simulink model "MotorGenerador_2016"  (Simulink 8.8)
settings: Solver=FixedStepAuto  StartTime=0.0  StopTime=inf  RelTol=1e-3  EnableMultiTasking=on
undefined symbols (not defined in the file or in its folder): sigbuilder_block
libraries: arduinolib x2, simulink x1
settings Model: Creator=Sergio  LastModifiedBy=Sergio  SimulationMode=external  ExtModeTrigDuration=2
settings DataIOCC: LimitDataPoints=off  SaveFormat=Dataset  SignalLoggingSaveFormat=Dataset
settings OptimizationCC: EnhancedBackFolding=on  PassReuseOutputArgsAs=Individual arguments  ZeroExternalMemoryAtStartup=off  ZeroInternalMemoryAtStartup=off  LifeSpan=auto  MaxStackSize=64
settings DebuggingCC: UnderspecifiedInitializationDetection=Simplified  MergeDetectMultiDrivingBlocksExec=error  ParameterTunabilityLossMsg=error  FcnCallInpInsideContextMsg=error  StateNameClashWarn=none  SFUnexpectedBacktrackingDiag=error  SFNoUnconditionalDefaultTransitionDiag=error  SFExecutionAtInitializationDiag=warning  SFMachineParentedDataDiag=error
settings HardwareCC: ProdBitPerInt=16  ProdBitPerPointer=16  ProdBitPerSizeT=16  ProdBitPerPtrDiffT=16  ProdIntDivRoundTo=Zero  ProdEndianess=LittleEndian  ProdWordSize=8  ProdHWDeviceType=Atmel->AVR
settings ModelReferenceCC: PropagateSignalLabelsOutOfModel=on
settings SFSimCC: SimUseLocalCustomCode=on
settings RTWCC: Description=Embedded Coder  SystemTargetFile=ert.tlc  HardwareBoard=Arduino Leonardo  TLCOptions=-aInlineSetEventsForThisBaseRateFcn=TLC_FALSE -aSuppressMultiTaskScheduler=TLC_FALSE -aRateBasedStepFcn=1  TemplateMakefile=ert_default_tmf  RTWUseLocalCustomCode=on  Toolchain=Arduino AVR  BuildConfiguration=Faster Runs
settings MATStruct: className=codertarget.tools.BuildHook  argsTopModelOnly=[]  excludedModels=[]  includeReferencedModels=on  includeTopModel=on  enabled=on  UseCoderTarget=[1.0]  TargetHardware=Arduino Leonardo  RTOS=Baremetal  Scheduler_interrupt_source=[0.0]  DataVersion=2016.02  Baudrate=115200  COMPort=codertarget.arduinobase.internal.getExternalModeMexArgs('Serial')  Verbose=[0.0]  IPAddress=codertarget.arduinobase.internal.getExternalModeMexArgs('Ethernet')  Port=17725  Configuration=Serial  COMPortBaud=115200  HostInterface=Simulink  signalBufferSize=[250.0]  Running=on  BuildAction=Build, load and run  DisableParallelBuild=[0.0]  ForceBuildStaticLibrary=[0.0]  Set_host_COM_port=Automatically  COM_port_number=1  Bootloader_COM_port=2  Enable_SimulinkIO=[1.0]  Enable_overrun_detection=[0.0]  Digital_output_to_set_on_overrun=13  Analog_input_reference_voltage=[0.0]  Serial0_baud_rate=9600  Serial1_baud_rate=9600  I2C0BusSpeedHz=100000  SPI_clock_out_frequency=4000  SPI_mode=Mode 0 - Clock Polarity 0, Clock Phase 0  SPI_bitorder=MSB first  SDSlaveSelect=[4.0]  CANChipSelect=[9.0]  Disable_DHCP_Ethernet=[0.0]  Local_ip_address=192.168.0.20  Local_mac_address=DE:AD:BE:EF:FE:ED  Wifi_Hardware=WiFi shield  Disable_DHCP_Wifi=[0.0]  Wifi_ip_address=192.168.1.20  Wifi_SSID=yourNetwork  Set_Wifi_Encryption=None  Wifi_WEP_key=D0D0DEADF00DABBADEAFBEADED  Wifi_WEP_key_index=0  Wifi_WPA_password=secretPassword  Wifi_ESP8266_HW_serial_port=Serial 1  Enable_CustomServer=0  IP_address=184.106.153.149  CANBusSpeed=500  CANOscillatorFrequency=16  InterruptPin=[2.0]  AllowAllFilter=[0.0]  Buffer0IDType=Normal  AcceptanceMask0_Nor=0  AcceptanceFilter0_Nor=255  AcceptanceFilter1_Nor=255  AcceptanceMask0_Ext=0  AcceptanceFilter0_Ext=255  AcceptanceFilter1_Ext=255  Buffer1IDType=Normal  AcceptanceMask1_Nor=0  AcceptanceFilter2_Nor=255  AcceptanceFilter3_Nor=255  AcceptanceFilter4_Nor=255  AcceptanceFilter5_Nor=255  AcceptanceMask1_Ext=0  AcceptanceFilter2_Ext=255  AcceptanceFilter3_Ext=255  AcceptanceFilter4_Ext=255  AcceptanceFilter5_Ext=255  Modbus_comms=RS485  Modbus_mode=Master  Modbus_slaveID=1  Modbus_configCoil=1  Modbus_CoilAddr=0  Modbus_CoilNum=1  Modbus_configInput=1  Modbus_InputAddr=0  Modbus_InputNum=1  Modbus_configHoldingReg=1  Modbus_HoldingRegAddr=0  Modbus_HoldingRegNum=1  Modbus_configInputReg=1  Modbus_InputRegAddr=0  Modbus_InputRegNum=1  Modbus_MasterTimeout=100  RS485_serial=Serial 1  RS485_baud=9600  RS485_Config=SERIAL_8N1  RS485_DEPin=8  RS485_REPin=9  EnableCodegen=[0.0]  AppLaunchButton=[]  enableCodegen=[0.0]  Codegen=[1.0]  Blockclass=codertarget.targetHiddenBlkInsert.internal.circularGauge  RegFcn=codertarget.arduinobase.blocks.registerDashboardBlk  ValidateFcn=codertarget.targetHiddenBlkInsert.internal.isDashboardBlockCodegenEnabled
settings CodeAppCC: ForceParamTrailComments=on  IgnoreCustomStorageClasses=off  OperatorAnnotations=on  SimulinkDataObjDesc=on  SFDataObjDesc=on  InsertBlockDesc=on
settings ERTTargetCC: SupportContinuousTime=on  SupportVariableSizeSignals=on  ExtMode=on  ExtModeTransport=5  ExtModeStaticAllocSize=250  ExtModeMexFile=ext_serial_win32_comm_leonardo  ExtModeMexArgs=0 14 115200
settings ConfigComp: CovMetricSettings=dwe  CovSaveCumulativeToWorkspaceVar=off  CovSaveSingleToWorkspaceVar=off  CovExternalEMLEnable=on

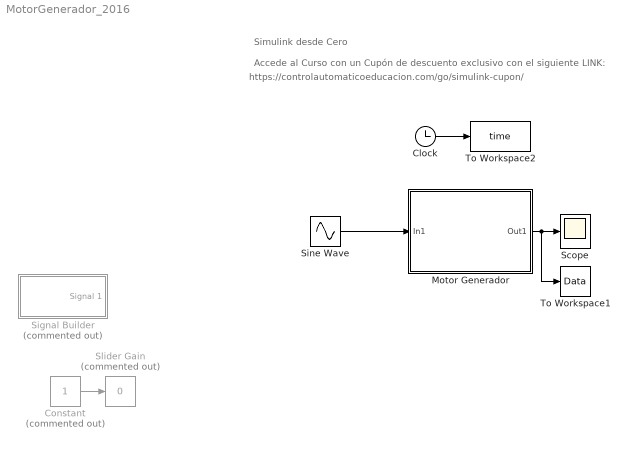
== system MotorGenerador_2016 ==
  note: https://controlautomaticoeducacion.com/go/simulink-cupon/
  note: Accede al Curso con un Cupón de descuento exclusivo con el siguiente LINK:
  note: Simulink desde Cero
  Clock : Clock
  Constant : Constant  Commented=on
  Motor Generador : Subsystem
  Scope : Scope
  Signal Builder : Subsystem  Tag=STV Subsys  Commented=on  LoadFcn=sigbuilder_block('load');  StartFcn=sigbuilder_block('start');  StopFcn=sigbuilder_block('stop');  ClipboardFcn=sigbuilder_block('clipboard');  mask(Sigbuilder block){tuvar=[0:10]}
      mask help: Simulink:masks:SigbuilderBlock_MD
      mask init:
      | if ~strcmp(get_param(bdroot(gcbh),'SimulationStatus'),'stopped') tuvar = sigbuilder_block('maskInit'); end
      settings: CopyFcn=sigbuilder_block('copy');  DeleteFcn=sigbuilder_block('delete');  ModelCloseFcn=sigbuilder_block('modelClose');  PreSaveFcn=sigbuilder_block('preSave');  PauseFcn=sigbuilder_block('pause');  ContinueFcn=sigbuilder_block('continue');  NameChangeFcn=sigbuilder_block('namechange');  OpenFcn=sigbuilder_block('open',[437.6 199.2 550.4 400 ]);  CloseFcn=sigbuilder_block('close');
      mask Display: plot(0, 0, 100, 100,[2, 2, 32, 32, 2], [68, 8, 8, 68, 68],[32, 2], [38, 38], [32, 19, 2],[53, 60, 44], [32, 17, 17, 2],[16, 16, 31, 31]);txt = getActiveGroup(gcbh);text(2, 100, txt,'verticalAlignment', 'top');
  Sine Wave : Sin  Bias=3  Frequency=0.1  SampleTime=0
  Slider Gain : simulink/Math Operations/Slider Gain  Commented=on  gain=0  low=0  high=5
  To Workspace1 : ToWorkspace  VariableName=Data  SampleTime=0.01
  To Workspace2 : ToWorkspace  VariableName=time  SampleTime=0.01
  wires:
  Constant/1 -> Slider Gain/1
  Clock/1 -> To Workspace2/1
  Sine Wave/1 -> Motor Generador/1(In1)
  Motor Generador/1(Out1) -> To Workspace1/1, Scope/1

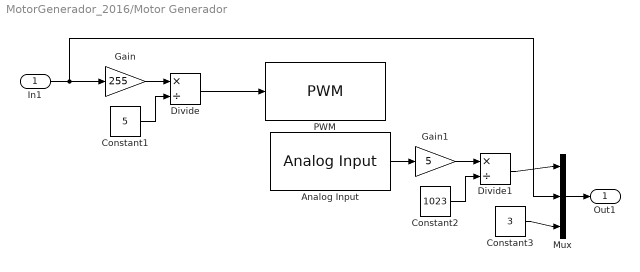
== system MotorGenerador_2016/Motor Generador ==
  In1 : Inport
  Analog Input : arduinolib/Analog Input  pinNumber=0  ReadResultsOnly=off  ConversionTriggerSource=Software  ExternalTriggerType=uint32( 0 )  OutputDataType=uint16  EnableConversionCompleteNotify=off  EnableOuputStatus=off  SampleTime=0.01  blockPlatform=arduino
  Constant1 : Constant  Value=5
  Constant2 : Constant  Value=1023
  Constant3 : Constant  Value=3
  Divide : Product  Inputs=*/
  Divide1 : Product  Inputs=*/
  Gain : Gain  Gain=255
  Gain1 : Gain  Gain=5
  Mux : Mux  Inputs=3
  PWM : arduinolib/PWM  pinNumber=10  frequencyType=Specify  desiredFrequency=490.2  achievableFrequency=490.1961
  Out1 : Outport
  wires:
  Constant1/1 -> Divide/2
  Gain1/1 -> Divide1/1
  Analog Input/1 -> Gain1/1
  Gain/1 -> Divide/1
  Constant2/1 -> Divide1/2
  Divide/1 -> PWM/1
  In1/1 -> Mux/2, Gain/1
  Divide1/1 -> Mux/1
  Mux/1 -> Out1/1
  Constant3/1 -> Mux/3

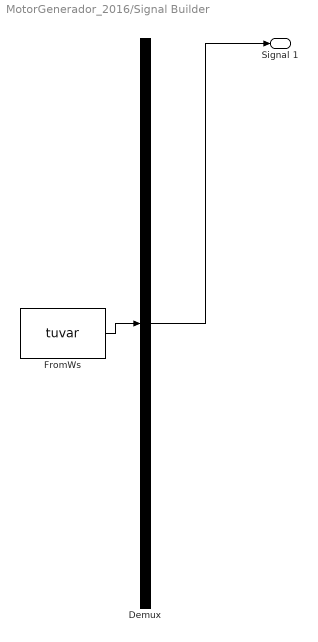
== system MotorGenerador_2016/Signal Builder ==
  Demux : Demux  Tag=STV Demux  Outputs=1
      settings: DisplayOption=none
  FromWs : FromWorkspace  Tag=STV FromWs  VariableName=tuvar  SigBuilderData=DataTag0  VnvData=DataTag1
      SigBuilderData=|
      | common.afterFinalStr = 'Extrapolate'
      | common.sampleTime = 0
      | dataSet.timeRange = [0 60]
      | dataSet.name = 'Group 1'
      | sbobj.Groups.Name = 'Group 1'
      | sbobj.Groups.Signals.Name = 'Signal 1'
      | sbobj.Groups.Signals.XData = [0 4 4 10 10 25 25 40 40 45 45 50 50 52 52 53 53 55 55 56 56 59 60]
      | sbobj.Groups.Signals.YData = [0 0 2 2 4 4 2 2 4 4 2 2 4 4 2 2 4 4 2 2 4 4 0]
      | sbobj.Groups.TimeRange = [0 60]
  Signal 1 : Outport  Tag=STV Outport
  wires:
  Demux/1 -> Signal 1/1
  FromWs/1 -> Demux/1
